simulink model "Team_2_Strategy"
settings: Solver=ode45  StartTime=0.0  StopTime=10.0  RelTol=1e-3
settings Model: Creator=smahapat  LastModifiedBy=user
settings SolverCC: ZeroCrossControl=DisableAll
settings DataIOCC: LimitDataPoints=on  SaveFormat=Array  SignalLoggingSaveFormat=ModelDataLogs  ReturnWorkspaceOutputs=off
settings OptimizationCC: InlineParams=on  ExpressionDepthLimit=2147483647  LifeSpan=inf  SimCompilerOptimization=Off
settings DebuggingCC: UnderspecifiedInitializationDetection=Classic  MergeDetectMultiDrivingBlocksExec=none  SolverPrmCheckMsg=warning  FcnCallInpInsideContextMsg=Use local settings  FrameProcessingCompatibilityMsg=warning  StateNameClashWarn=warning  SFUnexpectedBacktrackingDiag=warning  SFNoUnconditionalDefaultTransitionDiag=warning
settings HardwareCC: ProdBitPerPointer=32  ProdLargestAtomicFloat=None  ProdIntDivRoundTo=Undefined  ProdEndianess=Unspecified  ProdWordSize=32  ProdHWDeviceType=32-bit Generic
settings ModelReferenceCC: PropagateSignalLabelsOutOfModel=off
settings SFSimCC: SimUseLocalCustomCode=off  SimParseCustomCode=off
settings RTWCC: RTWUseLocalCustomCode=off  RTWCompilerOptimization=Off
settings CodeAppCC: CustomSymbolStrType=$N$R$M
settings GRTTargetCC: CodeReplacementLibrary=ANSI_C  GeneratePreprocessorConditionals=Disable all  CombineOutputUpdateFcns=off  CPPClassGenCompliant=off  GRTInterface=on

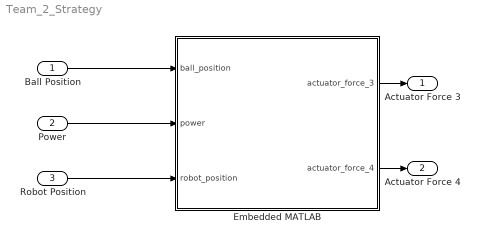
== system Team_2_Strategy ==
  Ball Position : Inport  PortDimensions=[2 1]
  Power : Inport  Port=2  PortDimensions=[4 1]  BusOutputAsStruct=on
  Robot Position : Inport  Port=3  PortDimensions=[8 1]  BusOutputAsStruct=on
  Embedded MATLAB : MATLAB Function  TreatAsAtomicUnit=on
  Actuator Force 3 : Outport
  Actuator Force 4 : Outport  Port=2
  wires:
  Embedded MATLAB/1(actuator_force_3) -> Actuator Force 3/1
  Power/1 -> Embedded MATLAB/2(power)
  Embedded MATLAB/2(actuator_force_4) -> Actuator Force 4/1
  Ball Position/1 -> Embedded MATLAB/1(ball_position)
  Robot Position/1 -> Embedded MATLAB/3(robot_position)

== matlab function Team_2_Strategy/Embedded MATLAB ==
  data: ball_position input; power input; robot_position input; actuator_force_3 output; actuator_force_4 output
function [actuator_force_3, actuator_force_4] = fcn( ball_position,power, robot_position)
%#eml

d3=(robot_position(5:6,1)-ball_position);
d4=(robot_position(7:8,1)-ball_position);
if dot(d3,d3)>2
   actuator_force_3=-133*d3;
else
   r3=(ball_position- [0;50]);
   actuator_force_3=-65*r3;
end
if dot(d4,d4)>2
   actuator_force_4=-123*d4;
else
   r4=(ball_position- [0;50]);
   actuator_force_4=-25*r4;
end
